simulink model "relay_nonlinearity"  (R2024a)
settings: Solver=FixedStepAuto  StartTime=0.0  StopTime=50  FixedStep=1e-6  RelTol=1e-3
settings Model: Creator=Lenovo  LastModifiedBy=Lenovo

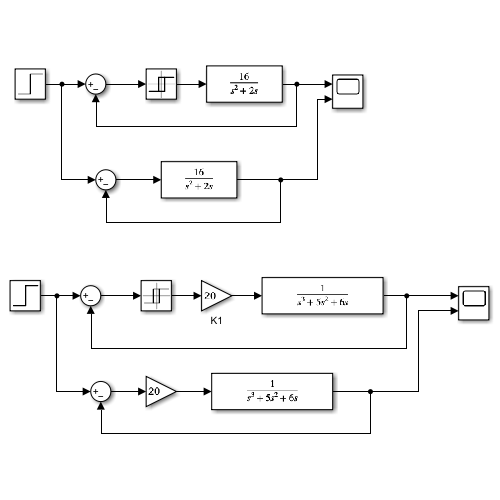
[thumbnail: Simulink's stored preview of the top-level diagram]
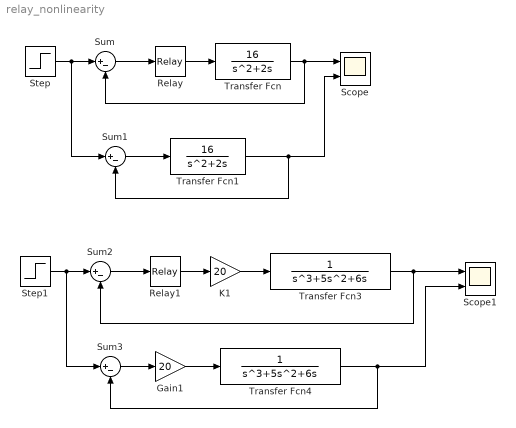
== system relay_nonlinearity ==
  Gain1 : Gain  Gain=20
  K1 : Gain  Gain=20
  Relay : Relay  OnSwitchValue=0  OffSwitchValue=0  OnOutputValue=0.5  OffOutputValue=-0.5
  Relay1 : Relay  OnSwitchValue=0  OffSwitchValue=0  OnOutputValue=0.5  OffOutputValue=-0.5
  Scope : Scope  NumInputPorts=2
  Scope1 : Scope  NumInputPorts=2
  Step : Step  SampleTime=0
  Step1 : Step  SampleTime=0
  Sum{,1..3} (4 alike) : Sum  Inputs=|+-
  Transfer Fcn : TransferFcn  Numerator=[16]  Denominator=[1 2 0]
  Transfer Fcn1 : TransferFcn  Numerator=[16]  Denominator=[1 2 0]
  Transfer Fcn3 : TransferFcn  Denominator=[1 5 6 0]
  Transfer Fcn4 : TransferFcn  Denominator=[1 5 6 0]
  wires:
  Sum/1 -> Relay/1
  Relay/1 -> Transfer Fcn/1
  Transfer Fcn/1 -> Sum/2, Scope/1
  Transfer Fcn1/1 -> Scope/2, Sum1/2
  Sum1/1 -> Transfer Fcn1/1
  Step/1 -> Sum1/1, Sum/1
  Step1/1 -> Sum2/1, Sum3/1
  Sum3/1 -> Gain1/1
  Transfer Fcn4/1 -> Sum3/2, Scope1/2
  Sum2/1 -> Relay1/1
  Relay1/1 -> K1/1
  Transfer Fcn3/1 -> Scope1/1, Sum2/2
  K1/1 -> Transfer Fcn3/1
  Gain1/1 -> Transfer Fcn4/1
